simulink model "wheel_mech"  (R2017b)
settings: Solver=ode23s  StartTime=0.0  StopTime=tfinal  FixedStep=dt  RelTol=1e-3
undefined symbols (not defined in the file): B_bearing, c1, c2, c3, dt, g, inits, Jw, Jy, M, mu_cal, N, r_eff, Reff
libraries: cstblocks x1
settings Model: Creator=Ehsan Arasteh  LastModifiedBy=ehsan
settings SolverCC: SolverJacobianMethodControl=FullAnalytical
settings OptimizationCC: LifeSpan=inf
settings DebuggingCC: SFExecutionAtInitializationDiag=none
settings CodeAppCC: StateflowObjectComments=on

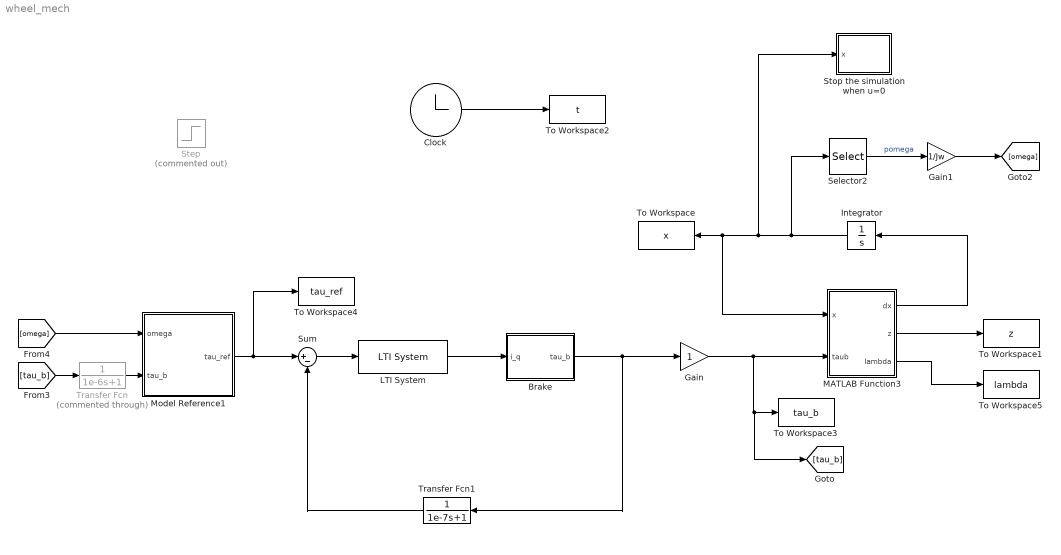
== system wheel_mech ==
  Brake : Subsystem
  Clock : Clock
  Gain : Gain
  Gain1 : Gain  Gain=1/Jw
  Integrator : Integrator  InitialCondition=inits
  LTI System : cstblocks/LTI System  sys=Gc_brake  IC=[]
  MATLAB Function3 : MATLAB Function  TreatAsAtomicUnit=on
  Model Reference1 : Subsystem
  Selector2 : Selector  InputPortWidth=2  IndexOptions=Index vector (dialog)  Indices=[1]  OutputSizes=1
  Step : Step  Commented=on  Time=0.5  After=1000  SampleTime=0
  Stop the simulation when u=0 : Subsystem
  Sum : Sum  Inputs=|+-
  To Workspace : ToWorkspace  VariableName=x  SampleTime=dt
  To Workspace1 : ToWorkspace  VariableName=z  SampleTime=dt
  To Workspace2 : ToWorkspace  VariableName=t  SampleTime=dt
  To Workspace3 : ToWorkspace  VariableName=tau_b  SampleTime=dt
  To Workspace4 : ToWorkspace  VariableName=tau_ref  SampleTime=dt
  To Workspace5 : ToWorkspace  VariableName=lambda  SampleTime=dt
  Transfer Fcn : TransferFcn  Commented=through  Denominator=[1e-6 1]
  Transfer Fcn1 : TransferFcn  Denominator=[1e-7 1]
  wires:
  MATLAB Function3/1(dx) -> Integrator/1
  MATLAB Function3/2(z) -> To Workspace1/1
  MATLAB Function3/3(lambda) -> To Workspace5/1
  Selector2/1 -> Gain1/1  "pomega"
  Integrator/1 -> Selector2/1, Stop the simulation when u=0/1(x), MATLAB Function3/1(x), To Workspace/1
  Clock/1 -> To Workspace2/1
  Gain1/1 -> [omega]
  Brake/1(tau_b) -> Transfer Fcn1/1, Gain/1
  Gain/1 -> [tau_b], To Workspace3/1, MATLAB Function3/2(taub)
  [tau_b] -> Transfer Fcn/1
  Model Reference1/1(tau_ref) -> To Workspace4/1, Sum/1
  [omega] -> Model Reference1/1(omega)
  Sum/1 -> LTI System/1
  LTI System/1 -> Brake/1(i_q)
  Transfer Fcn/1 -> Model Reference1/2(tau_b)
  Transfer Fcn1/1 -> Sum/2

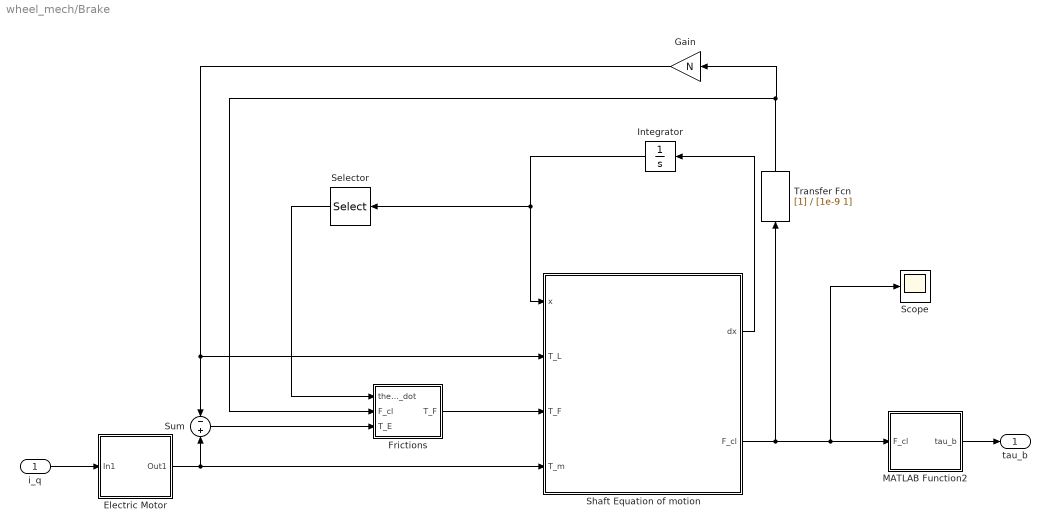
== system wheel_mech/Brake ==
  i_q : Inport
  Electric Motor : Subsystem
  Frictions : MATLAB Function  TreatAsAtomicUnit=on
  Gain : Gain  Gain=N
  Integrator : Integrator  InitialCondition=zeros(2,1)
  MATLAB Function2 : MATLAB Function  TreatAsAtomicUnit=on
  Scope : Scope
  Selector : Selector  InputPortWidth=2  IndexOptions=Index vector (dialog)  Indices=[1]  OutputSizes=1
  Shaft Equation of motion : MATLAB Function  TreatAsAtomicUnit=on
  Sum : Sum  Inputs=-|+
  Transfer Fcn : TransferFcn  Denominator=[1e-9 1]
  tau_b : Outport
  wires:
  MATLAB Function2/1(tau_b) -> tau_b/1
  Shaft Equation of motion/1(dx) -> Integrator/1
  Integrator/1 -> Shaft Equation of motion/1(x), Selector/1
  i_q/1 -> Electric Motor/1(In1)
  Electric Motor/1(Out1) -> Sum/2, Shaft Equation of motion/4(T_m)
  Sum/1 -> Frictions/3(T_E)
  Shaft Equation of motion/2(F_cl) -> Scope/1, MATLAB Function2/1(F_cl), Transfer Fcn/1
  Selector/1 -> Frictions/1(theta_dot)
  Gain/1 -> Shaft Equation of motion/2(T_L), Sum/1
  Transfer Fcn/1 -> Gain/1, Frictions/2(F_cl)
  Frictions/1(T_F) -> Shaft Equation of motion/3(T_F)

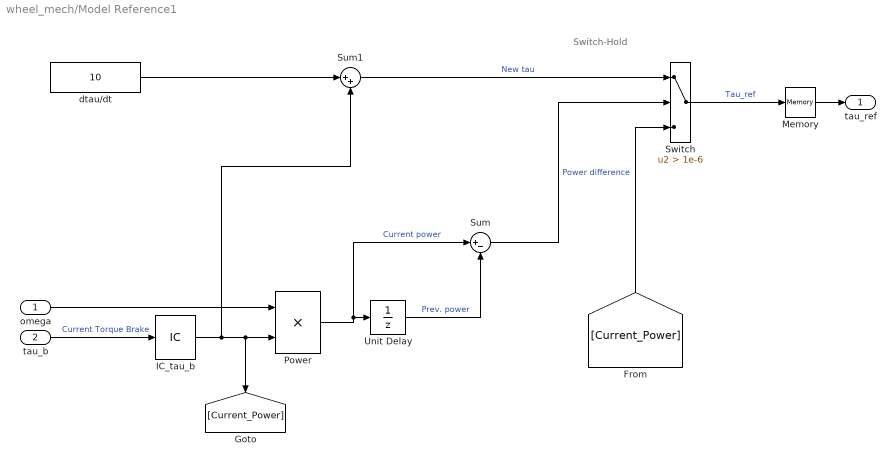
== system wheel_mech/Model Reference1 ==
  note: Switch-Hold
  omega : Inport
  tau_b : Inport  Port=2
  IC_tau_b : InitialCondition  Value=150
  Memory : Memory  InitialCondition=10
  Power : Product
  Sum : Sum  Inputs=|+-
  Sum1 : Sum  Inputs=|++
  Switch : Switch  Criteria=u2 > Threshold  Threshold=1e-6
  Unit Delay : UnitDelay  InitialCondition=150*inits(1)/Jy  SampleTime=2*dt
  dtau/dt : Constant  Value=10
  tau_ref : Outport
  wires:
  tau_b/1 -> IC_tau_b/1  "Current Torque Brake"
  dtau/dt/1 -> Sum1/1
  omega/1 -> Power/1
  Power/1 -> Unit Delay/1, Sum/1  "Current power"
  Unit Delay/1 -> Sum/2  "Prev. power"
  Switch/1 -> Memory/1  "Tau_ref"
  Sum/1 -> Switch/2  "Power difference"
  Sum1/1 -> Switch/1  "New tau"
  Memory/1 -> tau_ref/1
  IC_tau_b/1 -> Sum1/2, Power/2, [Current_Power]
  [Current_Power] -> Switch/3

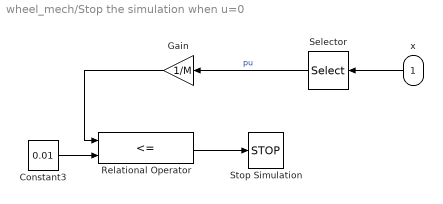
== system wheel_mech/Stop the simulation when u=0 ==
  x : Inport
  Constant3 : Constant  Value=0.01
  Gain : Gain  Gain=1/M
  Relational Operator : RelationalOperator  Operator=<=  OutDataTypeStr=boolean  RndMeth=Nearest
  Selector : Selector  InputPortWidth=2  IndexOptions=Index vector (dialog)  Indices=[2]  OutputSizes=1
  Stop Simulation : Stop
  wires:
  x/1 -> Selector/1
  Selector/1 -> Gain/1  "pu"
  Relational Operator/1 -> Stop Simulation/1
  Constant3/1 -> Relational Operator/2
  Gain/1 -> Relational Operator/1

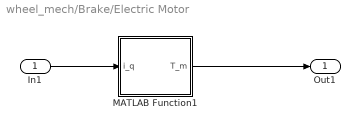
== system wheel_mech/Brake/Electric Motor ==
  In1 : Inport
  MATLAB Function1 : MATLAB Function  TreatAsAtomicUnit=on
  Out1 : Outport
  wires:
  In1/1 -> MATLAB Function1/1(i_q)
  MATLAB Function1/1(T_m) -> Out1/1

== matlab function wheel_mech/Brake/Shaft Equation of motion ==
  data: dx output; x input; T_L input; F_cl output; T_F input; T_m input; N parameter
function [dx,F_cl] = fcn(x,T_L,T_F,T_m,N)

% Parameters
J_m = 0.291e-3; % effective inertia


% States
theta_dot = x(1);
theta = x(2);


theta_2dot = (T_m-T_L-T_F)/J_m;
omega = theta_dot;


x_cal = N*theta; % Caliper position

x_cal = 1000*x_cal; %x_cal is in mm for the Calculation

if x_cal > 0.125
    F_cl = -7.23*x_cal^3+ 33.7*x_cal^2-3.97*x_cal;
else
    F_cl = 0.1295*x_cal;
end


F_cl = F_cl*1000; %F_cl is in kN


% kcal = 3.35e7;
% 
% x0 = 0.00015;
% if x_cal >= x0
%     F_cl = kcal*(x_cal-x0);
% else
%    F_cl = 0; 
% end

dx = [theta_2dot;omega];

== matlab function wheel_mech/MATLAB Function3 ==
  data: x input; dx output; taub input; Reff parameter; Jy parameter; z output; B_bearing parameter; M parameter; g parameter; c3 parameter; c2 parameter; c1 parameter; lambda output
function [dx, z, lambda]  = fcn(x, taub, Reff, Jy, B_bearing,  M, g, c3, c2, c1)


pw = x(1);
pu = x(2);

omega = pw./Jy;
u = pu./M;

lambda = (u-omega*Reff)./abs(max(u,omega*Reff));
mu = c1*(1-exp(-c2*lambda))-c3*lambda;

N = M*g;
Fb = mu.*N;


dpw = Fb*Reff - taub - B_bearing*omega;
dpu = -Fb;

if pw <= 0
   dpw = 0;
   pw = 0;
end

dx = [dpw;dpu];
z = [lambda; mu];

== matlab function wheel_mech/Brake/Electric Motor/MATLAB Function1 ==
  data: i_q input; T_m output
function T_m = fcn(i_q)

K_t = 0.0697; % Motor constant

T_m = K_t*i_q;


end

== matlab function wheel_mech/Brake/Frictions ==
  data: theta_dot input; T_F output; F_cl input; T_E input
function T_F = fcn(theta_dot,F_cl,T_E)

% Parameters
Ts = 0.0379;
G = 1.17e-5;
C = 0.0304;
D = 3.95e-4;
eps_f = 1e-9; % Karnopp friction threshold model


if abs(theta_dot) > eps_f
    T_F = D*theta_dot + (C+G*F_cl)* sign(theta_dot);
elseif abs(theta_dot) < eps_f && abs(T_E) < (Ts + G*F_cl)
    T_F = T_E;
else
    T_F = (Ts+G*F_cl)*sign(T_E);
end

== matlab function wheel_mech/Brake/MATLAB Function2 ==
  data: F_cl input; tau_b output; mu_cal parameter; r_eff parameter
function tau_b = fcn(F_cl,mu_cal, r_eff)


tau_b = 2*mu_cal*r_eff*F_cl;
